simulink model "ex7_v2"  (R2020a)
settings: Solver=VariableStepAuto  StartTime=0.0  StopTime=30  RelTol=1e-8
undefined symbols (not defined in the file): A, B, C, D, lambda, x01, x02
settings Model: Creator=Tomo  LastModifiedBy=Tomo

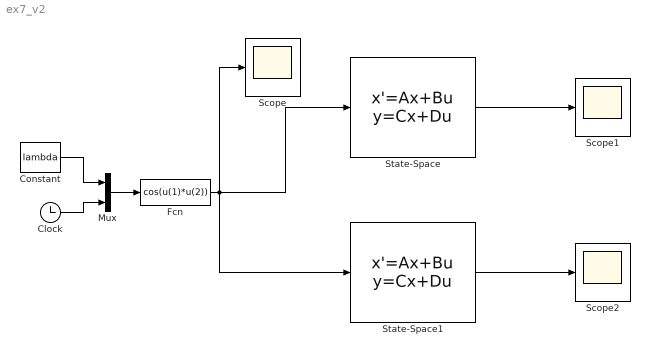
== system ex7_v2 ==
  Clock : Clock
  Constant : Constant  Value=lambda
  Fcn : Fcn  Expr=cos(u(1)*u(2))
  Mux : Mux  Inputs=2
  Scope : Scope
  Scope1 : Scope
  Scope2 : Scope
  State-Space : StateSpace  A=A  B=B  C=C  D=D  InitialCondition=x01
  State-Space1 : StateSpace  A=A  B=B  C=C  D=D  InitialCondition=x02
  wires:
  State-Space/1 -> Scope1/1
  State-Space1/1 -> Scope2/1
  Fcn/1 -> State-Space1/1, State-Space/1, Scope/1
  Constant/1 -> Mux/1
  Clock/1 -> Mux/2
  Mux/1 -> Fcn/1
